simulink model "System"  (R2019b)
settings: Solver=VariableStepAuto  StartTime=0.0  StopTime=10.0  RelTol=1e-3
settings Model: Creator=Lenovo  LastModifiedBy=Lenovo
settings OptimizationCC: DefaultParameterBehavior=Inlined

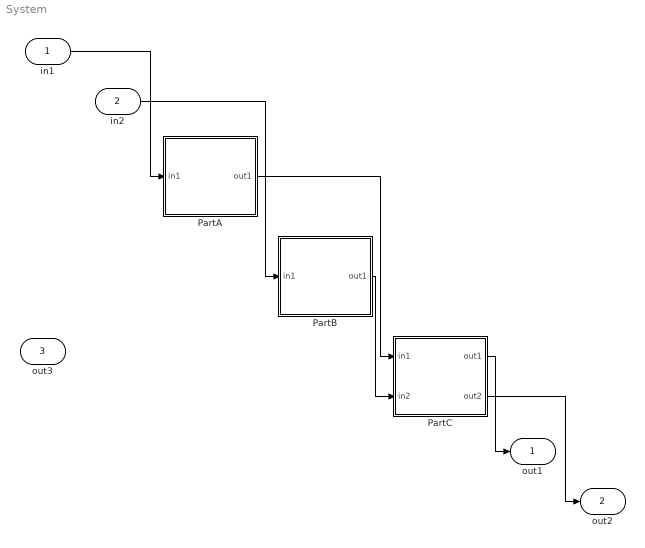
== system System ==
  in1 : Inport  OutDataTypeStr=double
  in2 : Inport  Port=2  OutDataTypeStr=int32
  PartA : Subsystem
  PartB : Subsystem
  PartC : Subsystem
  out1 : Outport  OutDataTypeStr=double
  out2 : Outport  Port=2  OutDataTypeStr=boolean
  out3 : Outport  Port=3  OutDataTypeStr=boolean
  wires:
  in1/1 -> PartA/1(in1)
  in2/1 -> PartB/1(in1)
  PartA/1(out1) -> PartC/1(in1)
  PartB/1(out1) -> PartC/2(in2)
  PartC/1(out1) -> out1/1
  PartC/2(out2) -> out2/1

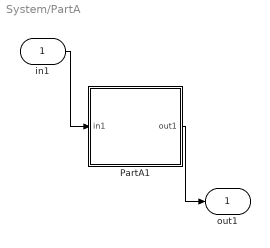
== system System/PartA ==
  in1 : Inport  OutDataTypeStr=double
  PartA1 : Subsystem
  out1 : Outport  OutDataTypeStr=double
  wires:
  in1/1 -> PartA1/1(in1)
  PartA1/1(out1) -> out1/1

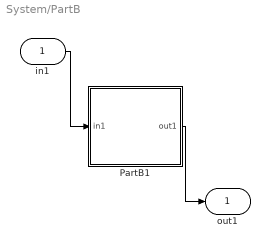
== system System/PartB ==
  in1 : Inport  OutDataTypeStr=int32
  PartB1 : Subsystem
  out1 : Outport  OutDataTypeStr=int32
  wires:
  in1/1 -> PartB1/1(in1)
  PartB1/1(out1) -> out1/1

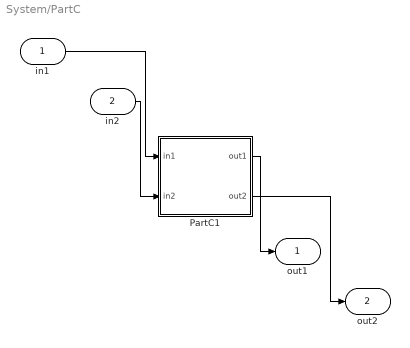
== system System/PartC ==
  in1 : Inport  OutDataTypeStr=double
  in2 : Inport  Port=2  OutDataTypeStr=int32
  PartC1 : Subsystem
  out1 : Outport  OutDataTypeStr=double
  out2 : Outport  Port=2  OutDataTypeStr=boolean
  wires:
  in1/1 -> PartC1/1(in1)
  in2/1 -> PartC1/2(in2)
  PartC1/1(out1) -> out1/1
  PartC1/2(out2) -> out2/1

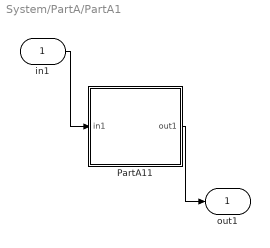
== system System/PartA/PartA1 ==
  in1 : Inport  OutDataTypeStr=double
  PartA11 : Subsystem
  out1 : Outport  OutDataTypeStr=double
  wires:
  in1/1 -> PartA11/1(in1)
  PartA11/1(out1) -> out1/1

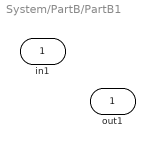
== system System/PartB/PartB1 ==
  in1 : Inport  OutDataTypeStr=int32
  out1 : Outport  OutDataTypeStr=int32

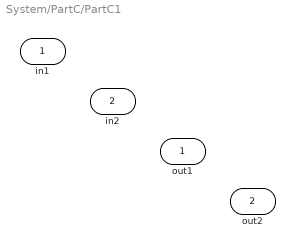
== system System/PartC/PartC1 ==
  in1 : Inport  OutDataTypeStr=double
  in2 : Inport  Port=2  OutDataTypeStr=int32
  out1 : Outport  OutDataTypeStr=double
  out2 : Outport  Port=2  OutDataTypeStr=boolean

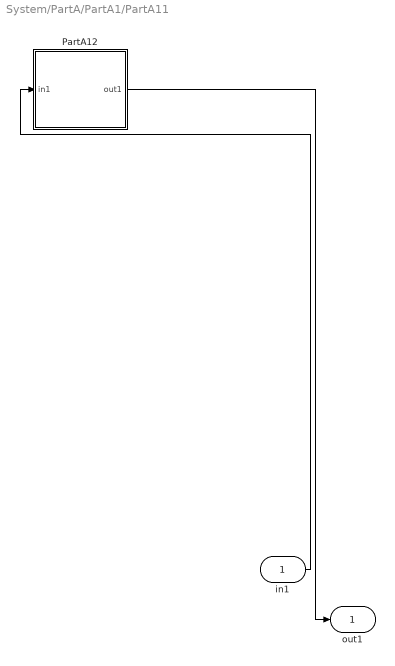
== system System/PartA/PartA1/PartA11 ==
  in1 : Inport  OutDataTypeStr=double
  PartA12 : Subsystem
  out1 : Outport  OutDataTypeStr=double
  wires:
  in1/1 -> PartA12/1(in1)
  PartA12/1(out1) -> out1/1

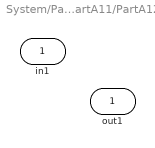
== system System/PartA/PartA1/PartA11/PartA12 ==
  in1 : Inport  OutDataTypeStr=double
  out1 : Outport  OutDataTypeStr=double
